simulink model "fig1_sim"  (R2014a)
settings: Solver=ode45  SolverMode=SingleTasking  StartTime=0.0  StopTime=30.0  RelTol=1e-3
undefined symbols (not defined in the file or in its folder): sigbuilder_block
settings Model: CovSFcnEnable=on  Creator=Katilv  LastModifiedBy=Hamidreza
settings OptimizationCC: BlockReduction=off  BooleanDataType=off
settings DebuggingCC: SaveWithParameterizedLinksMsg=none  UnderspecifiedInitializationDetection=Classic  SignalResolutionControl=TryResolveAllWithWarning  SolverPrmCheckMsg=none  StrictBusMsg=Warning
settings HardwareCC: TargetUnknown=on

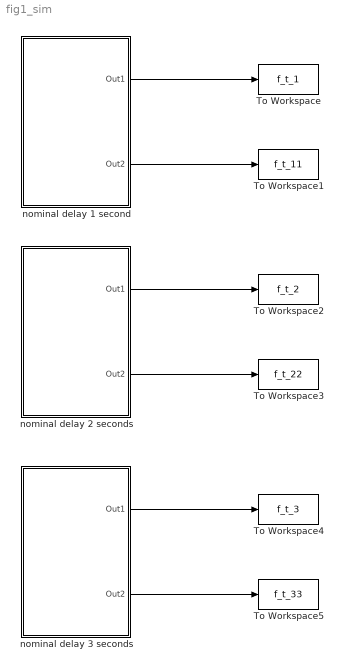
== system fig1_sim ==
  To Workspace : ToWorkspace  VariableName=f_t_1  SampleTime=-1
  To Workspace1 : ToWorkspace  VariableName=f_t_11  SampleTime=-1
  To Workspace2 : ToWorkspace  VariableName=f_t_2  SampleTime=-1
  To Workspace3 : ToWorkspace  VariableName=f_t_22  SampleTime=-1
  To Workspace4 : ToWorkspace  VariableName=f_t_3  SampleTime=-1
  To Workspace5 : ToWorkspace  VariableName=f_t_33  SampleTime=-1
  nominal delay 1 second : Subsystem
  nominal delay 2 seconds : Subsystem
  nominal delay 3 seconds : Subsystem
  wires:
  nominal delay 1 second/1(Out1) -> To Workspace/1
  nominal delay 1 second/2(Out2) -> To Workspace1/1
  nominal delay 2 seconds/2(Out2) -> To Workspace3/1
  nominal delay 2 seconds/1(Out1) -> To Workspace2/1
  nominal delay 3 seconds/1(Out1) -> To Workspace4/1
  nominal delay 3 seconds/2(Out2) -> To Workspace5/1

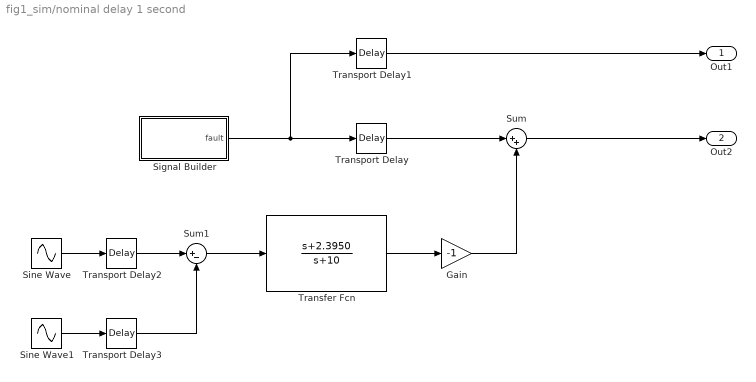
== system fig1_sim/nominal delay 1 second ==
  Gain : Gain  Gain=-1
  Signal Builder : Subsystem  Tag=STV Subsys  LoadFcn=sigbuilder_block('load');  StartFcn=sigbuilder_block('start');  StopFcn=sigbuilder_block('stop');  ClipboardFcn=sigbuilder_block('clipboard');  mask(Sigbuilder block){}
      mask help: Simulink:masks:SigbuilderBlock_MD
      mask init:
      | if ~strcmp(get_param(bdroot(gcbh),'SimulationStatus'),'stopped') tuvar = sigbuilder_block('maskInit'); end
      settings: CopyFcn=sigbuilder_block('copy');  DeleteFcn=sigbuilder_block('delete');  ModelCloseFcn=sigbuilder_block('modelClose');  PreSaveFcn=sigbuilder_block('preSave');  PauseFcn=sigbuilder_block('pause');  ContinueFcn=sigbuilder_block('continue');  NameChangeFcn=sigbuilder_block('namechange');  OpenFcn=sigbuilder_block('open',[192.75 153 550.5 359.25 ]);  CloseFcn=sigbuilder_block('close');
      mask Display: plot(0, 0, 100, 100,[2, 2, 32, 32, 2], [68, 8, 8, 68, 68],[32, 2], [38, 38], [32, 19, 2],[53, 60, 44], [32, 17, 17, 2],[16, 16, 31, 31]);txt = getActiveGroup(gcbh);text(2, 100, txt,'verticalAlignment', 'top');
  Sine Wave : Sin  Amplitude=0.5  Frequency=0.5  SampleTime=0
  Sine Wave1 : Sin  Amplitude=0.5  Frequency=0.5  SampleTime=0
  Sum : Sum  Inputs=|++
  Sum1 : Sum  Inputs=|+-
  Transfer Fcn : TransferFcn  Numerator=[1 2.3950]  Denominator=[1 10]
  Transport Delay : TransportDelay  DelayTime=1.1
  Transport Delay1 : TransportDelay
  Transport Delay2 : TransportDelay
  Transport Delay3 : TransportDelay  DelayTime=1.1
  Out1 : Outport
  Out2 : Outport  Port=2
  wires:
  Gain/1 -> Sum/2
  Transport Delay/1 -> Sum/1
  Sum/1 -> Out2/1
  Transport Delay3/1 -> Sum1/2
  Sine Wave1/1 -> Transport Delay3/1
  Sine Wave/1 -> Transport Delay2/1
  Transport Delay2/1 -> Sum1/1
  Sum1/1 -> Transfer Fcn/1
  Transfer Fcn/1 -> Gain/1
  Transport Delay1/1 -> Out1/1
  Signal Builder/1(fault) -> Transport Delay1/1, Transport Delay/1

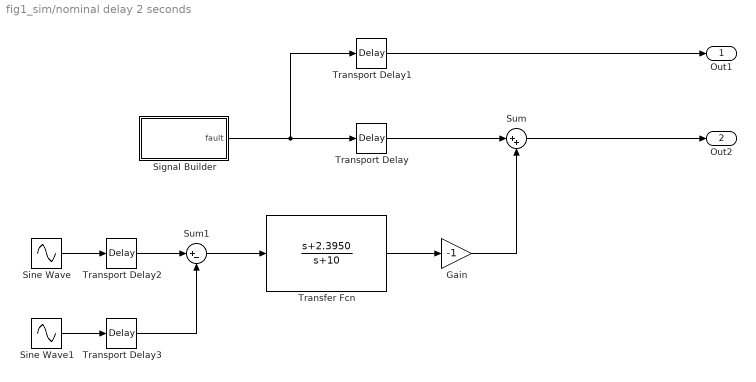
== system fig1_sim/nominal delay 2 seconds ==
  Gain : Gain  Gain=-1
  Signal Builder : Subsystem  Tag=STV Subsys  LoadFcn=sigbuilder_block('load');  StartFcn=sigbuilder_block('start');  StopFcn=sigbuilder_block('stop');  ClipboardFcn=sigbuilder_block('clipboard');  mask(Sigbuilder block){}
      mask help: Simulink:masks:SigbuilderBlock_MD
      mask init:
      | if ~strcmp(get_param(bdroot(gcbh),'SimulationStatus'),'stopped') tuvar = sigbuilder_block('maskInit'); end
      settings: CopyFcn=sigbuilder_block('copy');  DeleteFcn=sigbuilder_block('delete');  ModelCloseFcn=sigbuilder_block('modelClose');  PreSaveFcn=sigbuilder_block('preSave');  PauseFcn=sigbuilder_block('pause');  ContinueFcn=sigbuilder_block('continue');  NameChangeFcn=sigbuilder_block('namechange');  OpenFcn=sigbuilder_block('open',[192.75 153 550.5 359.25 ]);  CloseFcn=sigbuilder_block('close');
      mask Display: plot(0, 0, 100, 100,[2, 2, 32, 32, 2], [68, 8, 8, 68, 68],[32, 2], [38, 38], [32, 19, 2],[53, 60, 44], [32, 17, 17, 2],[16, 16, 31, 31]);txt = getActiveGroup(gcbh);text(2, 100, txt,'verticalAlignment', 'top');
  Sine Wave : Sin  Amplitude=0.5  Frequency=0.5  SampleTime=0
  Sine Wave1 : Sin  Amplitude=0.5  Frequency=0.5  SampleTime=0
  Sum : Sum  Inputs=|++
  Sum1 : Sum  Inputs=|+-
  Transfer Fcn : TransferFcn  Numerator=[1 2.3950]  Denominator=[1 10]
  Transport Delay : TransportDelay  DelayTime=2.2
  Transport Delay1 : TransportDelay  DelayTime=2
  Transport Delay2 : TransportDelay  DelayTime=2
  Transport Delay3 : TransportDelay  DelayTime=2.2
  Out1 : Outport
  Out2 : Outport  Port=2
  wires:
  Gain/1 -> Sum/2
  Transport Delay/1 -> Sum/1
  Sum/1 -> Out2/1
  Transport Delay3/1 -> Sum1/2
  Sine Wave1/1 -> Transport Delay3/1
  Sine Wave/1 -> Transport Delay2/1
  Transport Delay2/1 -> Sum1/1
  Sum1/1 -> Transfer Fcn/1
  Transfer Fcn/1 -> Gain/1
  Transport Delay1/1 -> Out1/1
  Signal Builder/1(fault) -> Transport Delay1/1, Transport Delay/1

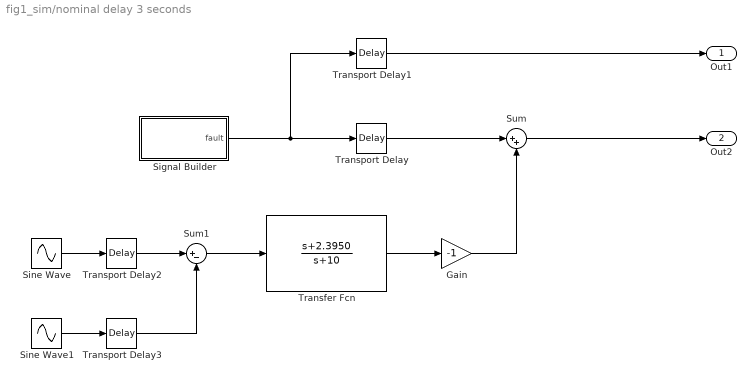
== system fig1_sim/nominal delay 3 seconds ==
  Gain : Gain  Gain=-1
  Signal Builder : Subsystem  Tag=STV Subsys  LoadFcn=sigbuilder_block('load');  StartFcn=sigbuilder_block('start');  StopFcn=sigbuilder_block('stop');  ClipboardFcn=sigbuilder_block('clipboard');  mask(Sigbuilder block){}
      mask help: Simulink:masks:SigbuilderBlock_MD
      mask init:
      | if ~strcmp(get_param(bdroot(gcbh),'SimulationStatus'),'stopped') tuvar = sigbuilder_block('maskInit'); end
      settings: CopyFcn=sigbuilder_block('copy');  DeleteFcn=sigbuilder_block('delete');  ModelCloseFcn=sigbuilder_block('modelClose');  PreSaveFcn=sigbuilder_block('preSave');  PauseFcn=sigbuilder_block('pause');  ContinueFcn=sigbuilder_block('continue');  NameChangeFcn=sigbuilder_block('namechange');  OpenFcn=sigbuilder_block('open',[192.75 153 550.5 359.25 ]);  CloseFcn=sigbuilder_block('close');
      mask Display: plot(0, 0, 100, 100,[2, 2, 32, 32, 2], [68, 8, 8, 68, 68],[32, 2], [38, 38], [32, 19, 2],[53, 60, 44], [32, 17, 17, 2],[16, 16, 31, 31]);txt = getActiveGroup(gcbh);text(2, 100, txt,'verticalAlignment', 'top');
  Sine Wave : Sin  Amplitude=0.5  Frequency=0.5  SampleTime=0
  Sine Wave1 : Sin  Amplitude=0.5  Frequency=0.5  SampleTime=0
  Sum : Sum  Inputs=|++
  Sum1 : Sum  Inputs=|+-
  Transfer Fcn : TransferFcn  Numerator=[1 2.3950]  Denominator=[1 10]
  Transport Delay : TransportDelay  DelayTime=3.3
  Transport Delay1 : TransportDelay  DelayTime=3
  Transport Delay2 : TransportDelay  DelayTime=3
  Transport Delay3 : TransportDelay  DelayTime=3.3
  Out1 : Outport
  Out2 : Outport  Port=2
  wires:
  Gain/1 -> Sum/2
  Transport Delay/1 -> Sum/1
  Sum/1 -> Out2/1
  Transport Delay3/1 -> Sum1/2
  Sine Wave1/1 -> Transport Delay3/1
  Sine Wave/1 -> Transport Delay2/1
  Transport Delay2/1 -> Sum1/1
  Sum1/1 -> Transfer Fcn/1
  Transfer Fcn/1 -> Gain/1
  Transport Delay1/1 -> Out1/1
  Signal Builder/1(fault) -> Transport Delay1/1, Transport Delay/1

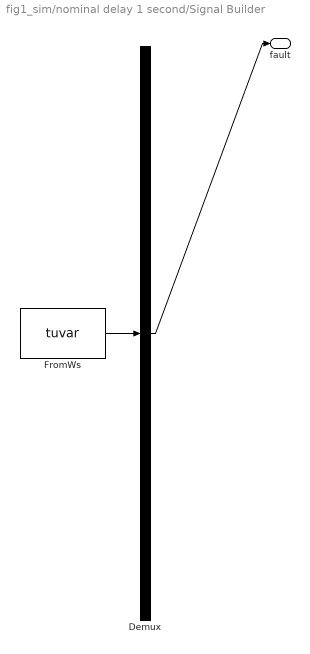
== system fig1_sim/nominal delay 1 second/Signal Builder ==
  Demux : Demux  Tag=STV Demux  Outputs=1
  FromWs : FromWorkspace  Tag=STV FromWs  VariableName=tuvar  SampleTime=0
      SigBuilderData=|
      | common.afterFinalStr = 'Extrapolate'
      | common.sampleTime = 0
      | dataSet.timeRange = [0 25]
      | dataSet.name = 'Group 1'
      | sbobj.Groups.Name = 'Group 1'
      | sbobj.Groups.Signals.Name = 'fault'
      | sbobj.Groups.Signals.XData = [0 5 10 15 25]
      | sbobj.Groups.Signals.YData = [0 0 1 0 0]
      | sbobj.Groups.TimeRange = [0 25]
  fault : Outport  Tag=STV Outport
  wires:
  FromWs/1 -> Demux/1
  Demux/1 -> fault/1

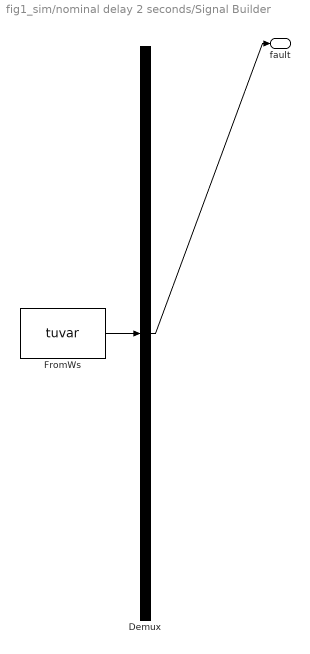
== system fig1_sim/nominal delay 2 seconds/Signal Builder ==
  Demux : Demux  Tag=STV Demux  Outputs=1
  FromWs : FromWorkspace  Tag=STV FromWs  VariableName=tuvar  SampleTime=0
      SigBuilderData=|
      | common.afterFinalStr = 'Extrapolate'
      | common.sampleTime = 0
      | dataSet.timeRange = [0 25]
      | dataSet.name = 'Group 1'
      | sbobj.Groups.Name = 'Group 1'
      | sbobj.Groups.Signals.Name = 'fault'
      | sbobj.Groups.Signals.XData = [0 5 10 15 25]
      | sbobj.Groups.Signals.YData = [0 0 1 0 0]
      | sbobj.Groups.TimeRange = [0 25]
  fault : Outport  Tag=STV Outport
  wires:
  FromWs/1 -> Demux/1
  Demux/1 -> fault/1

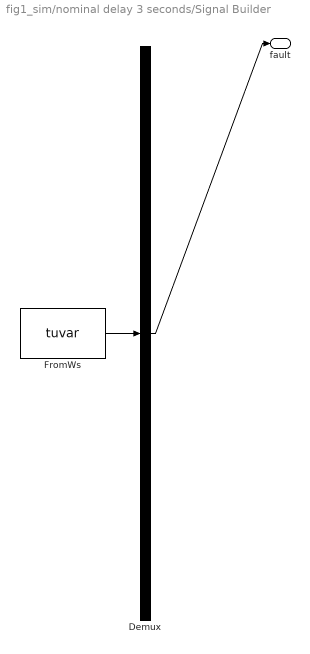
== system fig1_sim/nominal delay 3 seconds/Signal Builder ==
  Demux : Demux  Tag=STV Demux  Outputs=1
  FromWs : FromWorkspace  Tag=STV FromWs  VariableName=tuvar  SampleTime=0
      SigBuilderData=|
      | common.afterFinalStr = 'Extrapolate'
      | common.sampleTime = 0
      | dataSet.timeRange = [0 25]
      | dataSet.name = 'Group 1'
      | sbobj.Groups.Name = 'Group 1'
      | sbobj.Groups.Signals.Name = 'fault'
      | sbobj.Groups.Signals.XData = [0 5 10 15 25]
      | sbobj.Groups.Signals.YData = [0 0 1 0 0]
      | sbobj.Groups.TimeRange = [0 25]
  fault : Outport  Tag=STV Outport
  wires:
  FromWs/1 -> Demux/1
  Demux/1 -> fault/1
